simulink model "vectorized"  (R2017a)
settings: Solver=VariableStepAuto  StartTime=0.0  StopTime=10.0  RelTol=1e-3
settings Model: Creator=ptracton  LastModifiedBy=ptracton

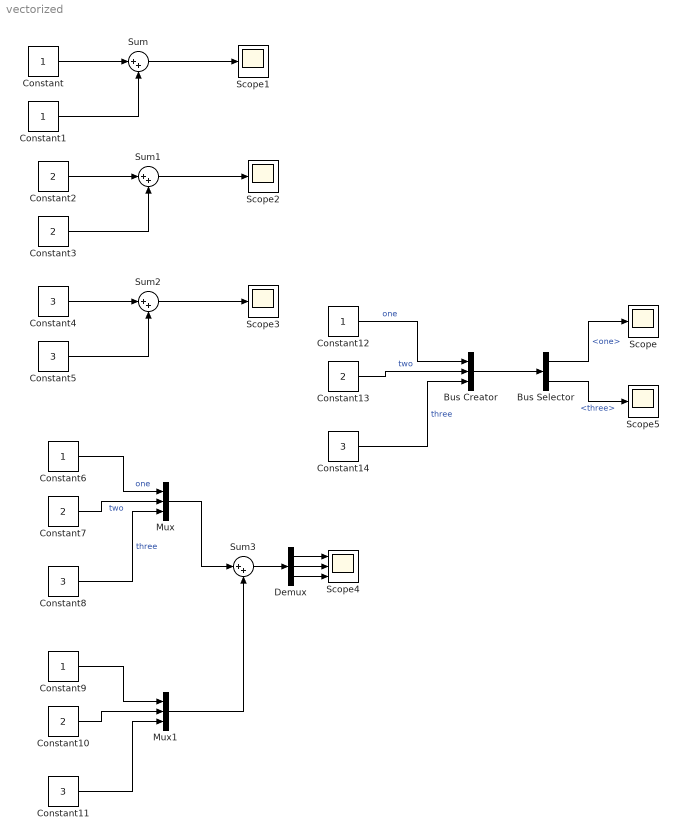
== system vectorized ==
  Bus Creator : BusCreator  Inputs=3
  Bus Selector : BusSelector  OutputSignals=one,three
  Constant{,1,6,9,12} (5 alike) : Constant
  Constant{2..3,7,10,13} (5 alike) : Constant  Value=2
  Constant{4..5,8,11,14} (5 alike) : Constant  Value=3
  Demux : Demux  Outputs=3
  Mux : Mux  Inputs=3
  Mux1 : Mux  Inputs=3
  Scope{,1..3,5} (5 alike) : Scope
  Scope4 : Scope  NumInputPorts=3
  Sum{,1..3} (4 alike) : Sum  Inputs=|++
  wires:
  Constant/1 -> Sum/1
  Sum/1 -> Scope1/1
  Constant1/1 -> Sum/2
  Sum1/1 -> Scope2/1
  Constant3/1 -> Sum1/2
  Constant2/1 -> Sum1/1
  Sum2/1 -> Scope3/1
  Constant5/1 -> Sum2/2
  Constant4/1 -> Sum2/1
  Constant6/1 -> Mux/1  "one"
  Constant7/1 -> Mux/2  "two"
  Constant8/1 -> Mux/3  "three"
  Constant11/1 -> Mux1/3
  Constant10/1 -> Mux1/2
  Constant9/1 -> Mux1/1
  Mux/1 -> Sum3/1
  Mux1/1 -> Sum3/2
  Sum3/1 -> Demux/1
  Demux/1 -> Scope4/1
  Demux/2 -> Scope4/2
  Demux/3 -> Scope4/3
  Constant14/1 -> Bus Creator/3  "three"
  Constant13/1 -> Bus Creator/2  "two"
  Constant12/1 -> Bus Creator/1  "one"
  Bus Creator/1 -> Bus Selector/1
  Bus Selector/1 -> Scope/1  "<one>"
  Bus Selector/2 -> Scope5/1  "<three>"
